simulink model "untitled"  (R2024a)
settings: Solver=VariableStepAuto  StartTime=0.0  StopTime=50  RelTol=1e-3
model workspace (MAT data in the model file):
  k1 = 1
  k2 = 1
  m = 1

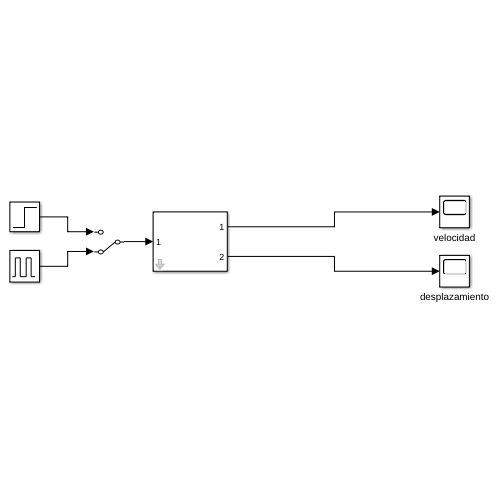
[thumbnail: Simulink's stored preview of the top-level diagram]
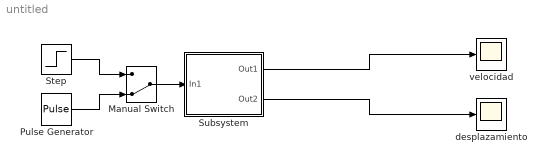
== system untitled ==
  Manual Switch : ManualSwitch  CurrentSetting=0
  Pulse Generator : DiscretePulseGenerator  PulseType=Time based  Period=10  PulseWidth=5
  Step : Step  SampleTime=0
  Subsystem : Subsystem  mask{m=1, k1=1, k2=1}
      mask prompts: m "Masa:"; k1 "Cte. Roce"; k2 "Cte. Resorte"
  desplazamiento : Scope
  velocidad : Scope
  wires:
  Step/1 -> Manual Switch/1
  Subsystem/1(Out1) -> velocidad/1
  Subsystem/2(Out2) -> desplazamiento/1
  Manual Switch/1 -> Subsystem/1(In1)
  Pulse Generator/1 -> Manual Switch/2

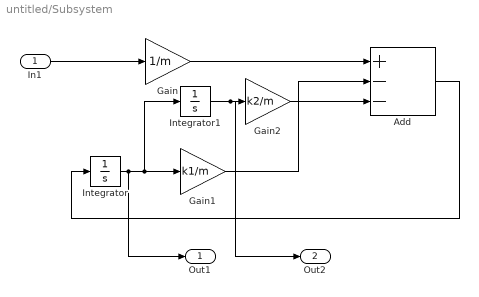
== system untitled/Subsystem ==
  In1 : Inport
  Add : Sum  Inputs=+--
  Gain : Gain  Gain=1/m
  Gain1 : Gain  Gain=k1/m
  Gain2 : Gain  Gain=k2/m
  Integrator : Integrator
  Integrator1 : Integrator
  Out1 : Outport
  Out2 : Outport  Port=2
  wires:
  Add/1 -> Integrator/1
  Gain/1 -> Add/1
  Gain1/1 -> Add/2
  Integrator1/1 -> Out2/1, Gain2/1
  In1/1 -> Gain/1
  Gain2/1 -> Add/3
  Integrator/1 -> Out1/1, Gain1/1, Integrator1/1
